simulink library "read_b"  (R2024b)
settings: Solver=VariableStepAuto  StartTime=0.0  StopTime=10.0  RelTol=1e-3
settings Model: Creator=eikel  LastModifiedBy=eikel

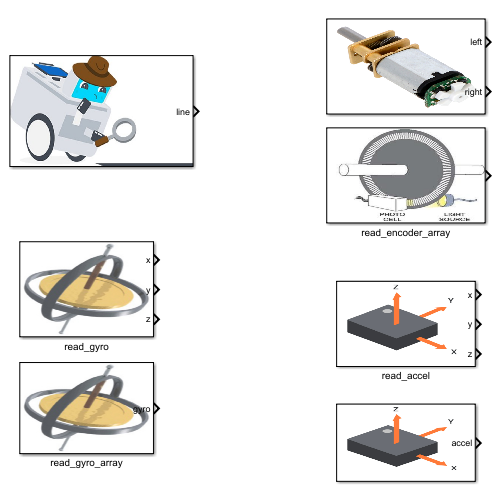
[thumbnail: Simulink's stored preview of the top-level diagram]
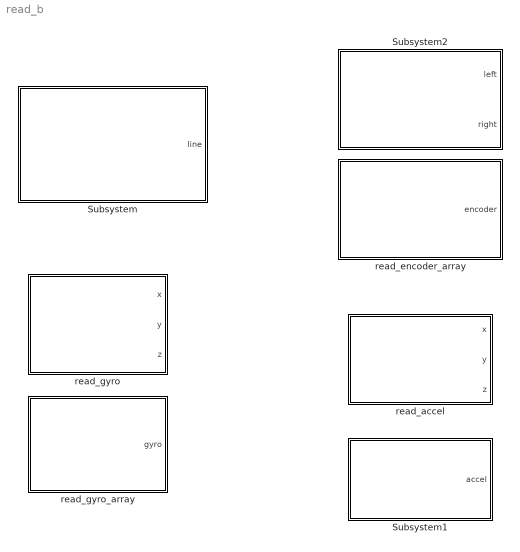
== system read_b ==
  Subsystem : Subsystem
      mask Display: image('lineDetector.jpg');
  Subsystem1 : Subsystem
      mask Display: image('accel.png');
  Subsystem2 : Subsystem
      mask Display: image('encoder_pololu.jpg');
  read_accel : Subsystem
      mask Display: image('accel.png');
  read_encoder_array : Subsystem
      mask Display: image('encoder_light.png');
  read_gyro : Subsystem
      mask Display: image('Gyroscope.jpg');
  read_gyro_array : Subsystem
      mask Display: image('Gyroscope.jpg');

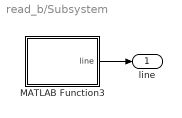
== system read_b/Subsystem ==
  MATLAB Function3 : MATLAB Function  TreatAsAtomicUnit=on
  line : Outport
  wires:
  MATLAB Function3/1(line) -> line/1

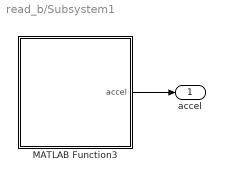
== system read_b/Subsystem1 ==
  MATLAB Function3 : MATLAB Function  TreatAsAtomicUnit=on
  accel : Outport
  wires:
  MATLAB Function3/1(accel) -> accel/1

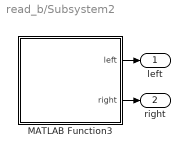
== system read_b/Subsystem2 ==
  MATLAB Function3 : MATLAB Function  TreatAsAtomicUnit=on
  left : Outport
  right : Outport  Port=2
  wires:
  MATLAB Function3/2(right) -> right/1
  MATLAB Function3/1(left) -> left/1

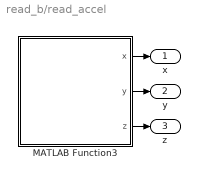
== system read_b/read_accel ==
  MATLAB Function3 : MATLAB Function  TreatAsAtomicUnit=on
  x : Outport
  y : Outport  Port=2
  z : Outport  Port=3
  wires:
  MATLAB Function3/3(z) -> z/1
  MATLAB Function3/2(y) -> y/1
  MATLAB Function3/1(x) -> x/1

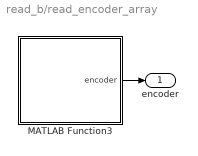
== system read_b/read_encoder_array ==
  MATLAB Function3 : MATLAB Function  TreatAsAtomicUnit=on
  encoder : Outport
  wires:
  MATLAB Function3/1(encoder) -> encoder/1

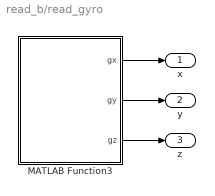
== system read_b/read_gyro ==
  MATLAB Function3 : MATLAB Function  TreatAsAtomicUnit=on
  x : Outport
  y : Outport  Port=2
  z : Outport  Port=3
  wires:
  MATLAB Function3/1(gx) -> x/1
  MATLAB Function3/2(gy) -> y/1
  MATLAB Function3/3(gz) -> z/1

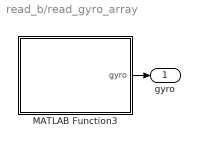
== system read_b/read_gyro_array ==
  MATLAB Function3 : MATLAB Function  TreatAsAtomicUnit=on
  gyro : Outport
  wires:
  MATLAB Function3/1(gyro) -> gyro/1

== matlab function read_b/read_gyro/MATLAB Function3 ==
  data: gx output; gy output; gz output
function [gx, gy, gz] = read_gyro()
    coder.extrinsic('get_gyro');
    gx = 0; gy = 0; gz = 0;
    [gx, gy, gz] = get_gyro();
end

== matlab function read_b/read_gyro_array/MATLAB Function3 ==
  data: gyro output
function gyro = read_gyro_vec()
    coder.extrinsic('get_gyro');
    gyro = zeros(1,3); % pre-alloc
    [x, y, z] = get_gyro();
    gyro = [x, y, z];
end

== matlab function read_b/read_accel/MATLAB Function3 ==
  data: x output; y output; z output
function [x, y, z] = read_accel_xyz()
    coder.extrinsic('get_accel_xyz');
    x = 0; y = 0; z = 0;
    [x, y, z] = get_accel_xyz();
end

== matlab function read_b/Subsystem1/MATLAB Function3 ==
  data: accel output
function accel = read_accel()
    coder.extrinsic('get_accel');
    accel = zeros(1,3); 
    [x, y, z] = get_accel();
    accel = [x, y, z];
end

== matlab function read_b/Subsystem2/MATLAB Function3 ==
  data: left output; right output
function [left, right]  = read_encoder()
    coder.extrinsic('get_encoder');
    left = 0; right = 0;
    [left, right] = get_encoder();
end

== matlab function read_b/read_encoder_array/MATLAB Function3 ==
  data: encoder output
function encoder = read_encoder()
    coder.extrinsic('get_encoder');
    encoder = zeros(1,2); % Forhåndsdefiner for Simulink sin del
    [left, right] = get_encoder();
    encoder = [left, right];
end

== matlab function read_b/Subsystem/MATLAB Function3 ==
  data: line output
function line = read_line()
    coder.extrinsic('get_line');  % merk: dette peikar på .m-fila di
    line =0;                         % initier output
    line_temp = get_line();            % kall den eksterne funksjonen
    if ~isnan(line_temp)
        line = line_temp;
    end
end
